simulink model "SIFT-Sysgen"  (R2013a)
settings: Solver=FixedStepDiscrete  SolverMode=SingleTasking  StartTime=0.0  StopTime=10.0  RelTol=1e-3
libraries: xbsIndex_r4 x365, xrbsImage_r4 x64
(part 2 of 10)

== system SIFT-Sysgen/Gaussian Filter3 ==
  In1 : Inport
  AddSub{,1..4} (5 alike) : xbsIndex_r4/AddSub  mode=Addition  use_carryin=off  use_carryout=off  en=off  latency=0  precision=Full  arith_type=Unsigned  n_bits=16  bin_pt=14  quantization=Truncate  overflow=Wrap  dbl_ovrd=off  use_behavioral_HDL=off  hw_selection=Fabric  pipelined=off  block_type=addsub
  Delay : xbsIndex_r4/Delay  rst=off  infoeditControl=Selection of Reset will increase slice count due to use of real FFs and instead of SRLs  en=off  latency=1  dbl_ovrd=off  reg_retiming=off  block_type=delay
  Subsystem : Subsystem
  Virtex Line Buffer : xrbsImage_r4/Virtex Line Buffer  buf_depth=720  cst=1
  Virtex2 Line Buffer : xrbsImage_r4/Virtex2 Line Buffer  buf_depth=720  cst=1
      link override Single Port RAM: block_version=8.2
  Virtex2 Line Buffer1 : xrbsImage_r4/Virtex2 Line Buffer  buf_depth=720  cst=1
      link override Single Port RAM: block_version=8.2
  Virtex2 Line Buffer2 : xrbsImage_r4/Virtex2 Line Buffer  buf_depth=720  cst=1
      link override Single Port RAM: block_version=8.2
  Out1 : Outport
  wires:
  In1/1 -> Subsystem/1(In1), Virtex Line Buffer/1
  Virtex Line Buffer/1 -> Virtex2 Line Buffer/1, Subsystem/2(In2)
  Virtex2 Line Buffer/1 -> Virtex2 Line Buffer1/1, Subsystem/3(In3)
  Virtex2 Line Buffer1/1 -> Subsystem/4(In4), Virtex2 Line Buffer2/1
  Virtex2 Line Buffer2/1 -> Subsystem/5(In5)
  Subsystem/1(Out1) -> AddSub/1
  Subsystem/2(Out2) -> AddSub/2
  Subsystem/3(Out3) -> AddSub1/1
  Subsystem/4(Out4) -> AddSub1/2
  Subsystem/5(Out5) -> AddSub2/1
  Subsystem/6(Out6) -> AddSub2/2
  AddSub/1 -> AddSub3/1
  AddSub1/1 -> AddSub3/2
  AddSub2/1 -> Delay/1
  Delay/1 -> AddSub4/2
  AddSub3/1 -> AddSub4/1
  AddSub4/1 -> Out1/1

== system SIFT-Sysgen/Gaussian Filter4 ==
  In1 : Inport
  AddSub{,1..4} (5 alike) : xbsIndex_r4/AddSub  mode=Addition  use_carryin=off  use_carryout=off  en=off  latency=0  precision=Full  arith_type=Unsigned  n_bits=16  bin_pt=14  quantization=Truncate  overflow=Wrap  dbl_ovrd=off  use_behavioral_HDL=off  hw_selection=Fabric  pipelined=off  block_type=addsub
  Delay : xbsIndex_r4/Delay  rst=off  infoeditControl=Selection of Reset will increase slice count due to use of real FFs and instead of SRLs  en=off  latency=1  dbl_ovrd=off  reg_retiming=off  block_type=delay
  Subsystem : Subsystem
  Virtex Line Buffer : xrbsImage_r4/Virtex Line Buffer  buf_depth=720  cst=1
  Virtex2 Line Buffer : xrbsImage_r4/Virtex2 Line Buffer  buf_depth=720  cst=1
      link override Single Port RAM: block_version=8.2
  Virtex2 Line Buffer1 : xrbsImage_r4/Virtex2 Line Buffer  buf_depth=720  cst=1
      link override Single Port RAM: block_version=8.2
  Virtex2 Line Buffer2 : xrbsImage_r4/Virtex2 Line Buffer  buf_depth=720  cst=1
      link override Single Port RAM: block_version=8.2
  Out1 : Outport
  wires:
  In1/1 -> Subsystem/1(In1), Virtex Line Buffer/1
  Virtex Line Buffer/1 -> Virtex2 Line Buffer/1, Subsystem/2(In2)
  Virtex2 Line Buffer/1 -> Virtex2 Line Buffer1/1, Subsystem/3(In3)
  Virtex2 Line Buffer1/1 -> Subsystem/4(In4), Virtex2 Line Buffer2/1
  Virtex2 Line Buffer2/1 -> Subsystem/5(In5)
  Subsystem/1(Out1) -> AddSub/1
  Subsystem/2(Out2) -> AddSub/2
  Subsystem/3(Out3) -> AddSub1/1
  Subsystem/4(Out4) -> AddSub1/2
  Subsystem/5(Out5) -> AddSub2/1
  Subsystem/6(Out6) -> AddSub2/2
  AddSub/1 -> AddSub3/1
  AddSub1/1 -> AddSub3/2
  AddSub2/1 -> Delay/1
  Delay/1 -> AddSub4/2
  AddSub3/1 -> AddSub4/1
  AddSub4/1 -> Out1/1

== system SIFT-Sysgen/Gaussian Filter5 ==
  In1 : Inport
  AddSub{,1..4} (5 alike) : xbsIndex_r4/AddSub  mode=Addition  use_carryin=off  use_carryout=off  en=off  latency=0  precision=Full  arith_type=Unsigned  n_bits=16  bin_pt=14  quantization=Truncate  overflow=Wrap  dbl_ovrd=off  use_behavioral_HDL=off  hw_selection=Fabric  pipelined=off  block_type=addsub
  Delay : xbsIndex_r4/Delay  rst=off  infoeditControl=Selection of Reset will increase slice count due to use of real FFs and instead of SRLs  en=off  latency=1  dbl_ovrd=off  reg_retiming=off  block_type=delay
  Subsystem : Subsystem
  Virtex Line Buffer : xrbsImage_r4/Virtex Line Buffer  buf_depth=720  cst=1
  Virtex2 Line Buffer : xrbsImage_r4/Virtex2 Line Buffer  buf_depth=720  cst=1
      link override Single Port RAM: block_version=8.2
  Virtex2 Line Buffer1 : xrbsImage_r4/Virtex2 Line Buffer  buf_depth=720  cst=1
      link override Single Port RAM: block_version=8.2
  Virtex2 Line Buffer2 : xrbsImage_r4/Virtex2 Line Buffer  buf_depth=720  cst=1
      link override Single Port RAM: block_version=8.2
  Out1 : Outport
  wires:
  In1/1 -> Subsystem/1(In1), Virtex Line Buffer/1
  Virtex Line Buffer/1 -> Virtex2 Line Buffer/1, Subsystem/2(In2)
  Virtex2 Line Buffer/1 -> Virtex2 Line Buffer1/1, Subsystem/3(In3)
  Virtex2 Line Buffer1/1 -> Subsystem/4(In4), Virtex2 Line Buffer2/1
  Virtex2 Line Buffer2/1 -> Subsystem/5(In5)
  Subsystem/1(Out1) -> AddSub/1
  Subsystem/2(Out2) -> AddSub/2
  Subsystem/3(Out3) -> AddSub1/1
  Subsystem/4(Out4) -> AddSub1/2
  Subsystem/5(Out5) -> AddSub2/1
  Subsystem/6(Out6) -> AddSub2/2
  AddSub/1 -> AddSub3/1
  AddSub1/1 -> AddSub3/2
  AddSub2/1 -> Delay/1
  Delay/1 -> AddSub4/2
  AddSub3/1 -> AddSub4/1
  AddSub4/1 -> Out1/1

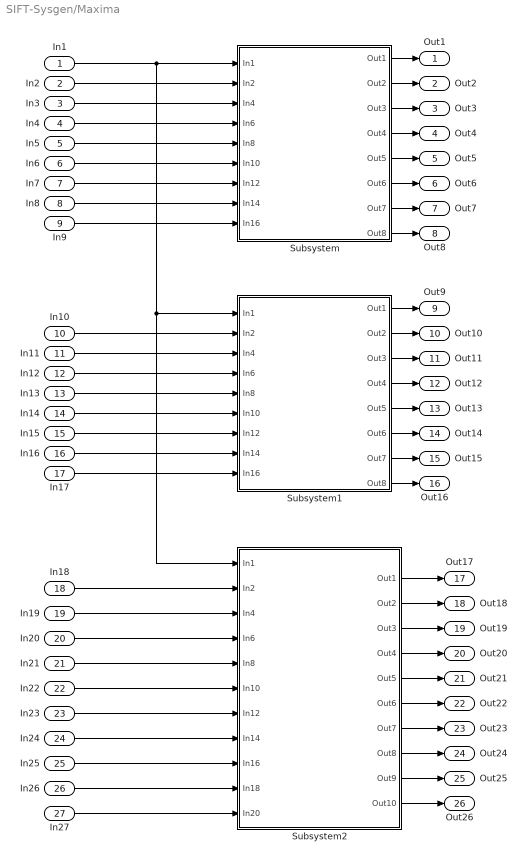
== system SIFT-Sysgen/Maxima ==
  In1 : Inport
  In2 : Inport  Port=2
  In3 : Inport  Port=3
  In4 : Inport  Port=4
  In5 : Inport  Port=5
  In6 : Inport  Port=6
  In7 : Inport  Port=7
  In8 : Inport  Port=8
  In9 : Inport  Port=9
  In10 : Inport  Port=10
  In11 : Inport  Port=11
  In12 : Inport  Port=12
  In13 : Inport  Port=13
  In14 : Inport  Port=14
  In15 : Inport  Port=15
  In16 : Inport  Port=16
  In17 : Inport  Port=17
  In18 : Inport  Port=18
  In19 : Inport  Port=19
  In20 : Inport  Port=20
  In21 : Inport  Port=21
  In22 : Inport  Port=22
  In23 : Inport  Port=23
  In24 : Inport  Port=24
  In25 : Inport  Port=25
  In26 : Inport  Port=26
  In27 : Inport  Port=27
  Subsystem : Subsystem
  Subsystem1 : Subsystem
  Subsystem2 : Subsystem
  Out1 : Outport
  Out2 : Outport  Port=2
  Out3 : Outport  Port=3
  Out4 : Outport  Port=4
  Out5 : Outport  Port=5
  Out6 : Outport  Port=6
  Out7 : Outport  Port=7
  Out8 : Outport  Port=8
  Out9 : Outport  Port=9
  Out10 : Outport  Port=10
  Out11 : Outport  Port=11
  Out12 : Outport  Port=12
  Out13 : Outport  Port=13
  Out14 : Outport  Port=14
  Out15 : Outport  Port=15
  Out16 : Outport  Port=16
  Out17 : Outport  Port=17
  Out18 : Outport  Port=18
  Out19 : Outport  Port=19
  Out20 : Outport  Port=20
  Out21 : Outport  Port=21
  Out22 : Outport  Port=22
  Out23 : Outport  Port=23
  Out24 : Outport  Port=24
  Out25 : Outport  Port=25
  Out26 : Outport  Port=26
  wires:
  In1/1 -> Subsystem/1(In1), Subsystem1/1(In1), Subsystem2/1(In1)
  In2/1 -> Subsystem/2(In2)
  In3/1 -> Subsystem/3(In4)
  In4/1 -> Subsystem/4(In6)
  In5/1 -> Subsystem/5(In8)
  In6/1 -> Subsystem/6(In10)
  In7/1 -> Subsystem/7(In12)
  In8/1 -> Subsystem/8(In14)
  In9/1 -> Subsystem/9(In16)
  In11/1 -> Subsystem1/3(In4)
  In12/1 -> Subsystem1/4(In6)
  In13/1 -> Subsystem1/5(In8)
  In14/1 -> Subsystem1/6(In10)
  In10/1 -> Subsystem1/2(In2)
  In15/1 -> Subsystem1/7(In12)
  In16/1 -> Subsystem1/8(In14)
  In17/1 -> Subsystem1/9(In16)
  In18/1 -> Subsystem2/2(In2)
  In19/1 -> Subsystem2/3(In4)
  In20/1 -> Subsystem2/4(In6)
  In21/1 -> Subsystem2/5(In8)
  In22/1 -> Subsystem2/6(In10)
  In23/1 -> Subsystem2/7(In12)
  In24/1 -> Subsystem2/8(In14)
  In25/1 -> Subsystem2/9(In16)
  Subsystem/1(Out1) -> Out1/1
  Subsystem/2(Out2) -> Out2/1
  Subsystem/3(Out3) -> Out3/1
  Subsystem/4(Out4) -> Out4/1
  Subsystem/5(Out5) -> Out5/1
  Subsystem/6(Out6) -> Out6/1
  Subsystem/7(Out7) -> Out7/1
  Subsystem/8(Out8) -> Out8/1
  Subsystem1/1(Out1) -> Out9/1
  Subsystem1/2(Out2) -> Out10/1
  Subsystem1/3(Out3) -> Out11/1
  Subsystem1/4(Out4) -> Out12/1
  Subsystem1/5(Out5) -> Out13/1
  Subsystem1/6(Out6) -> Out14/1
  Subsystem1/7(Out7) -> Out15/1
  Subsystem1/8(Out8) -> Out16/1
  Subsystem2/1(Out1) -> Out17/1
  Subsystem2/2(Out2) -> Out18/1
  Subsystem2/3(Out3) -> Out19/1
  Subsystem2/4(Out4) -> Out20/1
  Subsystem2/5(Out5) -> Out21/1
  Subsystem2/6(Out6) -> Out22/1
  Subsystem2/7(Out7) -> Out23/1
  Subsystem2/8(Out8) -> Out24/1
  In26/1 -> Subsystem2/10(In18)
  In27/1 -> Subsystem2/11(In20)
  Subsystem2/10(Out10) -> Out26/1
  Subsystem2/9(Out9) -> Out25/1

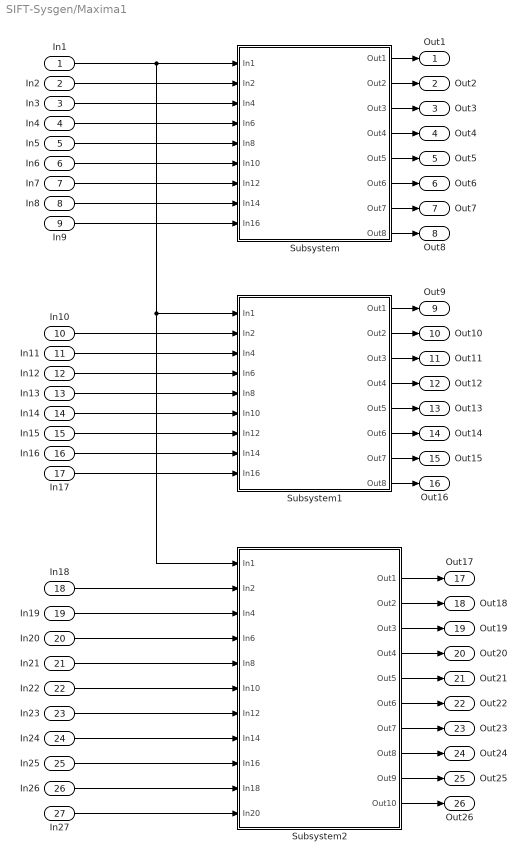
== system SIFT-Sysgen/Maxima1 ==
  In1 : Inport
  In2 : Inport  Port=2
  In3 : Inport  Port=3
  In4 : Inport  Port=4
  In5 : Inport  Port=5
  In6 : Inport  Port=6
  In7 : Inport  Port=7
  In8 : Inport  Port=8
  In9 : Inport  Port=9
  In10 : Inport  Port=10
  In11 : Inport  Port=11
  In12 : Inport  Port=12
  In13 : Inport  Port=13
  In14 : Inport  Port=14
  In15 : Inport  Port=15
  In16 : Inport  Port=16
  In17 : Inport  Port=17
  In18 : Inport  Port=18
  In19 : Inport  Port=19
  In20 : Inport  Port=20
  In21 : Inport  Port=21
  In22 : Inport  Port=22
  In23 : Inport  Port=23
  In24 : Inport  Port=24
  In25 : Inport  Port=25
  In26 : Inport  Port=26
  In27 : Inport  Port=27
  Subsystem : Subsystem
  Subsystem1 : Subsystem
  Subsystem2 : Subsystem
  Out1 : Outport
  Out2 : Outport  Port=2
  Out3 : Outport  Port=3
  Out4 : Outport  Port=4
  Out5 : Outport  Port=5
  Out6 : Outport  Port=6
  Out7 : Outport  Port=7
  Out8 : Outport  Port=8
  Out9 : Outport  Port=9
  Out10 : Outport  Port=10
  Out11 : Outport  Port=11
  Out12 : Outport  Port=12
  Out13 : Outport  Port=13
  Out14 : Outport  Port=14
  Out15 : Outport  Port=15
  Out16 : Outport  Port=16
  Out17 : Outport  Port=17
  Out18 : Outport  Port=18
  Out19 : Outport  Port=19
  Out20 : Outport  Port=20
  Out21 : Outport  Port=21
  Out22 : Outport  Port=22
  Out23 : Outport  Port=23
  Out24 : Outport  Port=24
  Out25 : Outport  Port=25
  Out26 : Outport  Port=26
  wires:
  In1/1 -> Subsystem/1(In1), Subsystem1/1(In1), Subsystem2/1(In1)
  In2/1 -> Subsystem/2(In2)
  In3/1 -> Subsystem/3(In4)
  In4/1 -> Subsystem/4(In6)
  In5/1 -> Subsystem/5(In8)
  In6/1 -> Subsystem/6(In10)
  In7/1 -> Subsystem/7(In12)
  In8/1 -> Subsystem/8(In14)
  In9/1 -> Subsystem/9(In16)
  In11/1 -> Subsystem1/3(In4)
  In12/1 -> Subsystem1/4(In6)
  In13/1 -> Subsystem1/5(In8)
  In14/1 -> Subsystem1/6(In10)
  In10/1 -> Subsystem1/2(In2)
  In15/1 -> Subsystem1/7(In12)
  In16/1 -> Subsystem1/8(In14)
  In17/1 -> Subsystem1/9(In16)
  In18/1 -> Subsystem2/2(In2)
  In19/1 -> Subsystem2/3(In4)
  In20/1 -> Subsystem2/4(In6)
  In21/1 -> Subsystem2/5(In8)
  In22/1 -> Subsystem2/6(In10)
  In23/1 -> Subsystem2/7(In12)
  In24/1 -> Subsystem2/8(In14)
  In25/1 -> Subsystem2/9(In16)
  Subsystem/1(Out1) -> Out1/1
  Subsystem/2(Out2) -> Out2/1
  Subsystem/3(Out3) -> Out3/1
  Subsystem/4(Out4) -> Out4/1
  Subsystem/5(Out5) -> Out5/1
  Subsystem/6(Out6) -> Out6/1
  Subsystem/7(Out7) -> Out7/1
  Subsystem/8(Out8) -> Out8/1
  Subsystem1/1(Out1) -> Out9/1
  Subsystem1/2(Out2) -> Out10/1
  Subsystem1/3(Out3) -> Out11/1
  Subsystem1/4(Out4) -> Out12/1
  Subsystem1/5(Out5) -> Out13/1
  Subsystem1/6(Out6) -> Out14/1
  Subsystem1/7(Out7) -> Out15/1
  Subsystem1/8(Out8) -> Out16/1
  Subsystem2/1(Out1) -> Out17/1
  Subsystem2/2(Out2) -> Out18/1
  Subsystem2/3(Out3) -> Out19/1
  Subsystem2/4(Out4) -> Out20/1
  Subsystem2/5(Out5) -> Out21/1
  Subsystem2/6(Out6) -> Out22/1
  Subsystem2/7(Out7) -> Out23/1
  Subsystem2/8(Out8) -> Out24/1
  In26/1 -> Subsystem2/10(In18)
  In27/1 -> Subsystem2/11(In20)
  Subsystem2/10(Out10) -> Out26/1
  Subsystem2/9(Out9) -> Out25/1

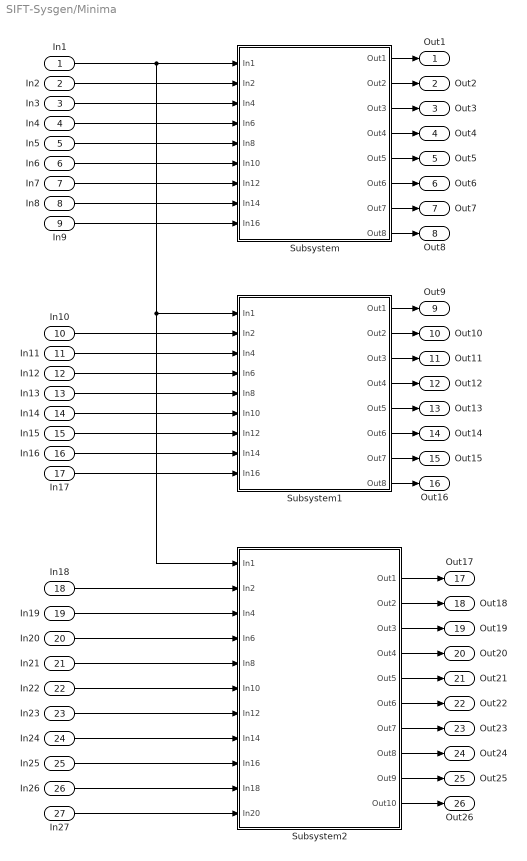
== system SIFT-Sysgen/Minima ==
  In1 : Inport
  In2 : Inport  Port=2
  In3 : Inport  Port=3
  In4 : Inport  Port=4
  In5 : Inport  Port=5
  In6 : Inport  Port=6
  In7 : Inport  Port=7
  In8 : Inport  Port=8
  In9 : Inport  Port=9
  In10 : Inport  Port=10
  In11 : Inport  Port=11
  In12 : Inport  Port=12
  In13 : Inport  Port=13
  In14 : Inport  Port=14
  In15 : Inport  Port=15
  In16 : Inport  Port=16
  In17 : Inport  Port=17
  In18 : Inport  Port=18
  In19 : Inport  Port=19
  In20 : Inport  Port=20
  In21 : Inport  Port=21
  In22 : Inport  Port=22
  In23 : Inport  Port=23
  In24 : Inport  Port=24
  In25 : Inport  Port=25
  In26 : Inport  Port=26
  In27 : Inport  Port=27
  Subsystem : Subsystem
  Subsystem1 : Subsystem
  Subsystem2 : Subsystem
  Out1 : Outport
  Out2 : Outport  Port=2
  Out3 : Outport  Port=3
  Out4 : Outport  Port=4
  Out5 : Outport  Port=5
  Out6 : Outport  Port=6
  Out7 : Outport  Port=7
  Out8 : Outport  Port=8
  Out9 : Outport  Port=9
  Out10 : Outport  Port=10
  Out11 : Outport  Port=11
  Out12 : Outport  Port=12
  Out13 : Outport  Port=13
  Out14 : Outport  Port=14
  Out15 : Outport  Port=15
  Out16 : Outport  Port=16
  Out17 : Outport  Port=17
  Out18 : Outport  Port=18
  Out19 : Outport  Port=19
  Out20 : Outport  Port=20
  Out21 : Outport  Port=21
  Out22 : Outport  Port=22
  Out23 : Outport  Port=23
  Out24 : Outport  Port=24
  Out25 : Outport  Port=25
  Out26 : Outport  Port=26
  wires:
  In1/1 -> Subsystem/1(In1), Subsystem1/1(In1), Subsystem2/1(In1)
  In2/1 -> Subsystem/2(In2)
  In3/1 -> Subsystem/3(In4)
  In4/1 -> Subsystem/4(In6)
  In5/1 -> Subsystem/5(In8)
  In6/1 -> Subsystem/6(In10)
  In7/1 -> Subsystem/7(In12)
  In8/1 -> Subsystem/8(In14)
  In9/1 -> Subsystem/9(In16)
  In11/1 -> Subsystem1/3(In4)
  In12/1 -> Subsystem1/4(In6)
  In13/1 -> Subsystem1/5(In8)
  In14/1 -> Subsystem1/6(In10)
  In10/1 -> Subsystem1/2(In2)
  In15/1 -> Subsystem1/7(In12)
  In16/1 -> Subsystem1/8(In14)
  In17/1 -> Subsystem1/9(In16)
  In18/1 -> Subsystem2/2(In2)
  In19/1 -> Subsystem2/3(In4)
  In20/1 -> Subsystem2/4(In6)
  In21/1 -> Subsystem2/5(In8)
  In22/1 -> Subsystem2/6(In10)
  In23/1 -> Subsystem2/7(In12)
  In24/1 -> Subsystem2/8(In14)
  In25/1 -> Subsystem2/9(In16)
  Subsystem/1(Out1) -> Out1/1
  Subsystem/2(Out2) -> Out2/1
  Subsystem/3(Out3) -> Out3/1
  Subsystem/4(Out4) -> Out4/1
  Subsystem/5(Out5) -> Out5/1
  Subsystem/6(Out6) -> Out6/1
  Subsystem/7(Out7) -> Out7/1
  Subsystem/8(Out8) -> Out8/1
  Subsystem1/1(Out1) -> Out9/1
  Subsystem1/2(Out2) -> Out10/1
  Subsystem1/3(Out3) -> Out11/1
  Subsystem1/4(Out4) -> Out12/1
  Subsystem1/5(Out5) -> Out13/1
  Subsystem1/6(Out6) -> Out14/1
  Subsystem1/7(Out7) -> Out15/1
  Subsystem1/8(Out8) -> Out16/1
  Subsystem2/1(Out1) -> Out17/1
  Subsystem2/2(Out2) -> Out18/1
  Subsystem2/3(Out3) -> Out19/1
  Subsystem2/4(Out4) -> Out20/1
  Subsystem2/5(Out5) -> Out21/1
  Subsystem2/6(Out6) -> Out22/1
  Subsystem2/7(Out7) -> Out23/1
  Subsystem2/8(Out8) -> Out24/1
  In26/1 -> Subsystem2/10(In18)
  In27/1 -> Subsystem2/11(In20)
  Subsystem2/10(Out10) -> Out26/1
  Subsystem2/9(Out9) -> Out25/1

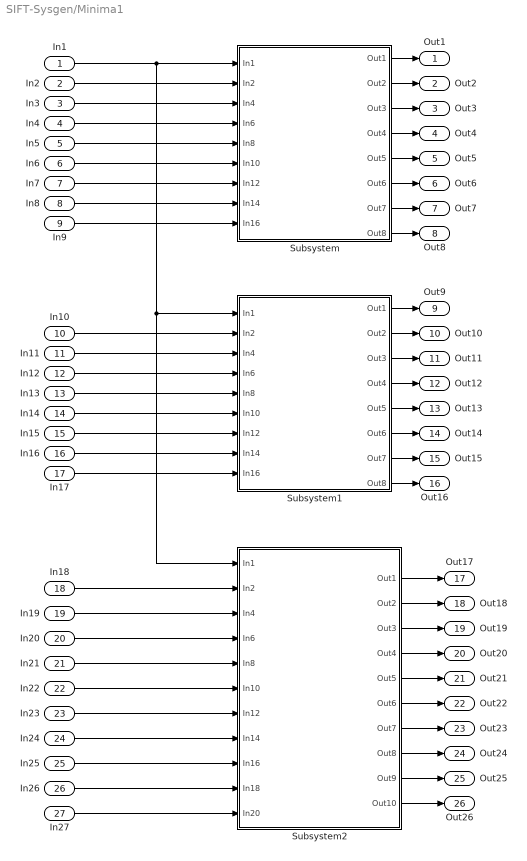
== system SIFT-Sysgen/Minima1 ==
  In1 : Inport
  In2 : Inport  Port=2
  In3 : Inport  Port=3
  In4 : Inport  Port=4
  In5 : Inport  Port=5
  In6 : Inport  Port=6
  In7 : Inport  Port=7
  In8 : Inport  Port=8
  In9 : Inport  Port=9
  In10 : Inport  Port=10
  In11 : Inport  Port=11
  In12 : Inport  Port=12
  In13 : Inport  Port=13
  In14 : Inport  Port=14
  In15 : Inport  Port=15
  In16 : Inport  Port=16
  In17 : Inport  Port=17
  In18 : Inport  Port=18
  In19 : Inport  Port=19
  In20 : Inport  Port=20
  In21 : Inport  Port=21
  In22 : Inport  Port=22
  In23 : Inport  Port=23
  In24 : Inport  Port=24
  In25 : Inport  Port=25
  In26 : Inport  Port=26
  In27 : Inport  Port=27
  Subsystem : Subsystem
  Subsystem1 : Subsystem
  Subsystem2 : Subsystem
  Out1 : Outport
  Out2 : Outport  Port=2
  Out3 : Outport  Port=3
  Out4 : Outport  Port=4
  Out5 : Outport  Port=5
  Out6 : Outport  Port=6
  Out7 : Outport  Port=7
  Out8 : Outport  Port=8
  Out9 : Outport  Port=9
  Out10 : Outport  Port=10
  Out11 : Outport  Port=11
  Out12 : Outport  Port=12
  Out13 : Outport  Port=13
  Out14 : Outport  Port=14
  Out15 : Outport  Port=15
  Out16 : Outport  Port=16
  Out17 : Outport  Port=17
  Out18 : Outport  Port=18
  Out19 : Outport  Port=19
  Out20 : Outport  Port=20
  Out21 : Outport  Port=21
  Out22 : Outport  Port=22
  Out23 : Outport  Port=23
  Out24 : Outport  Port=24
  Out25 : Outport  Port=25
  Out26 : Outport  Port=26
  wires:
  In1/1 -> Subsystem/1(In1), Subsystem1/1(In1), Subsystem2/1(In1)
  In2/1 -> Subsystem/2(In2)
  In3/1 -> Subsystem/3(In4)
  In4/1 -> Subsystem/4(In6)
  In5/1 -> Subsystem/5(In8)
  In6/1 -> Subsystem/6(In10)
  In7/1 -> Subsystem/7(In12)
  In8/1 -> Subsystem/8(In14)
  In9/1 -> Subsystem/9(In16)
  In11/1 -> Subsystem1/3(In4)
  In12/1 -> Subsystem1/4(In6)
  In13/1 -> Subsystem1/5(In8)
  In14/1 -> Subsystem1/6(In10)
  In10/1 -> Subsystem1/2(In2)
  In15/1 -> Subsystem1/7(In12)
  In16/1 -> Subsystem1/8(In14)
  In17/1 -> Subsystem1/9(In16)
  In18/1 -> Subsystem2/2(In2)
  In19/1 -> Subsystem2/3(In4)
  In20/1 -> Subsystem2/4(In6)
  In21/1 -> Subsystem2/5(In8)
  In22/1 -> Subsystem2/6(In10)
  In23/1 -> Subsystem2/7(In12)
  In24/1 -> Subsystem2/8(In14)
  In25/1 -> Subsystem2/9(In16)
  Subsystem/1(Out1) -> Out1/1
  Subsystem/2(Out2) -> Out2/1
  Subsystem/3(Out3) -> Out3/1
  Subsystem/4(Out4) -> Out4/1
  Subsystem/5(Out5) -> Out5/1
  Subsystem/6(Out6) -> Out6/1
  Subsystem/7(Out7) -> Out7/1
  Subsystem/8(Out8) -> Out8/1
  Subsystem1/1(Out1) -> Out9/1
  Subsystem1/2(Out2) -> Out10/1
  Subsystem1/3(Out3) -> Out11/1
  Subsystem1/4(Out4) -> Out12/1
  Subsystem1/5(Out5) -> Out13/1
  Subsystem1/6(Out6) -> Out14/1
  Subsystem1/7(Out7) -> Out15/1
  Subsystem1/8(Out8) -> Out16/1
  Subsystem2/1(Out1) -> Out17/1
  Subsystem2/2(Out2) -> Out18/1
  Subsystem2/3(Out3) -> Out19/1
  Subsystem2/4(Out4) -> Out20/1
  Subsystem2/5(Out5) -> Out21/1
  Subsystem2/6(Out6) -> Out22/1
  Subsystem2/7(Out7) -> Out23/1
  Subsystem2/8(Out8) -> Out24/1
  In26/1 -> Subsystem2/10(In18)
  In27/1 -> Subsystem2/11(In20)
  Subsystem2/10(Out10) -> Out26/1
  Subsystem2/9(Out9) -> Out25/1
